simulink library "abc_dq_lib_2011"  (Simulink 7.8)
settings: Solver=ode45  StartTime=0.0  StopTime=10.0  RelTol=1e-3
settings Model: Creator=CH24070  LastModifiedBy=ma25949

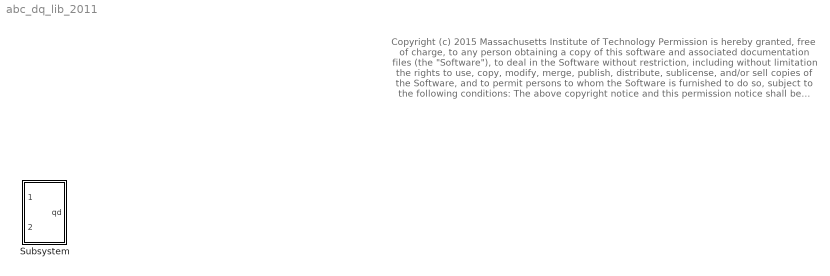
== system abc_dq_lib_2011 ==
  note: Copyright (c) 2015 Massachusetts Institute of Technology
      | Permission is hereby granted, free of charge, to any person obtaining a copy of this software and associated documentation files (the "Software"), to deal in the Software without restriction, including without limitation the rights to use, copy, modify, merge, publish, distribute, sublicense, and/or sell copies of the Software, and to permit persons to whom the Software is furnished to do so, subject to the following conditions:
      |
      | The above copyright notice and this permission notice shall be included in all copies or substantial portions of the Software.
      |
      | THE SOFTWARE IS PROVIDED "AS IS", WITHOUT WARRANTY OF ANY KIND, EXPRESS OR IMPLIED, INCLUDING BUT NOT LIMITED TO THE WARRANTIES OF MERCHANTABILITY, FITNESS FOR A PARTICULAR PURPOSE AND NONINFRINGEMENT. IN NO EVENT SHALL THE AUTHORS OR COPYRIGHT HOLDERS BE LIABLE FOR ANY CLAIM,
      | DAMAGES OR OTHER LIABILITY, WHETHER IN AN ACTION OF CONTRACT, TORT OR OTHERWISE, ARISING FROM, OUT OF OR IN CONNECTION WITH THE SOFTWARE OR THE USE OR OTHER DEALINGS IN THE SOFTWARE.
  Subsystem : Subsystem

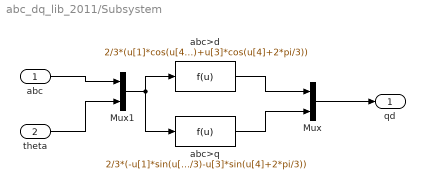
== system abc_dq_lib_2011/Subsystem ==
  abc : Inport  OutDataTypeStr=double  PortDimensions=3
  theta : Inport  Port=2  OutDataTypeStr=double  PortDimensions=1
  Mux : Mux  Inputs=2
  Mux1 : Mux  Inputs=2
  abc>d : Fcn  Expr=2/3*(u[1]*cos(u[4])+u[2]*cos(u[4]-2*pi/3)+u[3]*cos(u[4]+2*pi/3))
  abc>q : Fcn  Expr=2/3*(-u[1]*sin(u[4])-u[2]*sin(u[4]-2*pi/3)-u[3]*sin(u[4]+2*pi/3))
  qd : Outport  OutDataTypeStr=double  PortDimensions=2
  wires:
  Mux1/1 -> abc>q/1, abc>d/1
  Mux/1 -> qd/1
  abc>d/1 -> Mux/1
  abc>q/1 -> Mux/2
  theta/1 -> Mux1/2
  abc/1 -> Mux1/1
